simulink model "bicycle_model"  (R2018b)
settings: Solver=FixedStepAuto  StartTime=0.0  StopTime=10  FixedStep=0.001  RelTol=1e-3
values from neighbouring files (symbols this model uses):
  a = 1.8    [bicycle_coefficient_formula.m]    (also in bicycle_coefficient_roadcar.m = 1.1; formulacar_params.mat; roadcar_params.mat = 1.1)
  A = 1.25    [bicycle_coefficient_formula.m]    (also in bicycle_coefficient_roadcar.m = 1.8; formulacar_params.mat; roadcar_params.mat = 1.8)
  a1F = -1e-5    (= -1e-05)    [bicycle_coefficient_formula.m]    (also in bicycle_coefficient_roadcar.m; formulacar_params.mat; roadcar_params.mat)
  a1R = -1e-5    (= -1e-05)    [bicycle_coefficient_formula.m]    (also in bicycle_coefficient_roadcar.m; formulacar_params.mat; roadcar_params.mat)
  a2F = 1.25    [bicycle_coefficient_formula.m]    (also in bicycle_coefficient_roadcar.m = 0.95; formulacar_params.mat; roadcar_params.mat = 0.95)
  a2R = 1.25    [bicycle_coefficient_formula.m]    (also in bicycle_coefficient_roadcar.m = 0.95; formulacar_params.mat; roadcar_params.mat = 0.95)
  b = L-a    (= 1.7)    [bicycle_coefficient_formula.m]    (also in bicycle_coefficient_roadcar.m; formulacar_params.mat; roadcar_params.mat)
  BF = 0.2719    [bicycle_coefficient_formula.m]    (also in bicycle_coefficient_roadcar.m = 0.0813; formulacar_params.mat; roadcar_params.mat = 0.0813)
  BR = 0.3609    [bicycle_coefficient_formula.m]    (also in bicycle_coefficient_roadcar.m = 0.0925; formulacar_params.mat; roadcar_params.mat = 0.0925)
  CF = 1.8391    [bicycle_coefficient_formula.m]    (also in bicycle_coefficient_roadcar.m = 1.2947; formulacar_params.mat; roadcar_params.mat = 1.2947)
  CR = 1.7631    [bicycle_coefficient_formula.m]    (also in bicycle_coefficient_roadcar.m = 1.2617; formulacar_params.mat; roadcar_params.mat = 1.2617)
  cz = 1    [bicycle_coefficient_formula.m]    (also in bicycle_coefficient_roadcar.m = 0; formulacar_params.mat; roadcar_params.mat = 0)
  EF = -2.5276    [bicycle_coefficient_formula.m]    (also in bicycle_coefficient_roadcar.m = -8.3966; formulacar_params.mat; roadcar_params.mat = -8.3966)
  ER = -1.989    [bicycle_coefficient_formula.m]    (also in bicycle_coefficient_roadcar.m = -8.7012; formulacar_params.mat; roadcar_params.mat = -8.7012)
  g = 9.81    [bicycle_coefficient_formula.m]    (also in bicycle_coefficient_roadcar.m; formulacar_params.mat; roadcar_params.mat)
  I = 1500    [bicycle_coefficient_formula.m]    (also in bicycle_coefficient_roadcar.m = 3500; formulacar_params.mat; roadcar_params.mat = 3500)
  input = 1    [bicycle_script.m]    (also in formulacar_params.mat = 0; roadcar_params.mat = 0)
  L = 3.5    [bicycle_coefficient_formula.m]    (also in bicycle_coefficient_roadcar.m = 2.8; formulacar_params.mat; roadcar_params.mat = 2.8)
  m = 850    [bicycle_coefficient_formula.m]    (also in bicycle_coefficient_roadcar.m = 1650; formulacar_params.mat; roadcar_params.mat = 1650)
  rho = 1.225    [bicycle_coefficient_formula.m]    (also in bicycle_coefficient_roadcar.m; formulacar_params.mat; roadcar_params.mat)
  SA = 11    [bicycle_coefficient_formula.m]    (also in bicycle_coefficient_roadcar.m = 18; formulacar_params.mat; roadcar_params.mat = 18)
  slope = 2    [bicycle_coefficient_formula.m]    (also in bicycle_coefficient_roadcar.m; formulacar_params.mat; roadcar_params.mat)
  SR = 10    [bicycle_coefficient_formula.m]    (also in bicycle_coefficient_roadcar.m = 20; formulacar_params.mat; roadcar_params.mat = 20)
  V = 120    [bicycle_coefficient_formula.m]    (also in bicycle_coefficient_roadcar.m; formulacar_params.mat; roadcar_params.mat)
libraries: simulink_extras x5, simulink x1
settings Model: Creator=Cassio.Freitas  LastModifiedBy=Cassio.Freitas

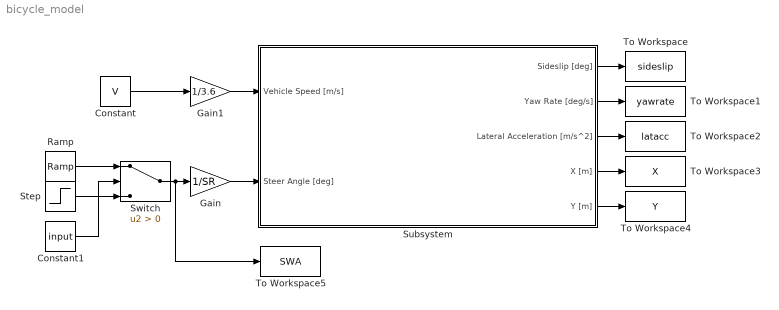
== system bicycle_model ==
  Constant : Constant  Value=V
  Constant1 : Constant  Value=input  SampleTime=0.01
  Gain : Gain  Gain=1/SR
  Gain1 : Gain  Gain=1/3.6
  Ramp : simulink/Sources/Ramp  slope=slope  start=0  InitialOutput=0
  Step : Step  Time=3  After=SA  SampleTime=0.001
  Subsystem : Subsystem
  Switch : Switch  Criteria=u2 > Threshold
  To Workspace : ToWorkspace  VariableName=sideslip  SaveFormat=Timeseries  SampleTime=-1
  To Workspace1 : ToWorkspace  VariableName=yawrate  SaveFormat=Timeseries  SampleTime=-1
  To Workspace2 : ToWorkspace  VariableName=latacc  SaveFormat=Timeseries  SampleTime=-1
  To Workspace3 : ToWorkspace  VariableName=X  SaveFormat=Timeseries  SampleTime=-1
  To Workspace4 : ToWorkspace  VariableName=Y  SaveFormat=Timeseries  SampleTime=-1
  To Workspace5 : ToWorkspace  VariableName=SWA  SaveFormat=Timeseries  SampleTime=-1
  wires:
  Subsystem/1(Sideslip [deg]) -> To Workspace/1
  Subsystem/2(Yaw Rate [deg/s]) -> To Workspace1/1
  Subsystem/3(Lateral Acceleration [m/s^2]) -> To Workspace2/1
  Subsystem/4(X [m]) -> To Workspace3/1
  Subsystem/5(Y [m]) -> To Workspace4/1
  Gain/1 -> Subsystem/2(Steer Angle [deg])
  Gain1/1 -> Subsystem/1(Vehicle Speed [m/s])
  Constant/1 -> Gain1/1
  Switch/1 -> To Workspace5/1, Gain/1
  Step/1 -> Switch/3
  Ramp/1 -> Switch/1
  Constant1/1 -> Switch/2

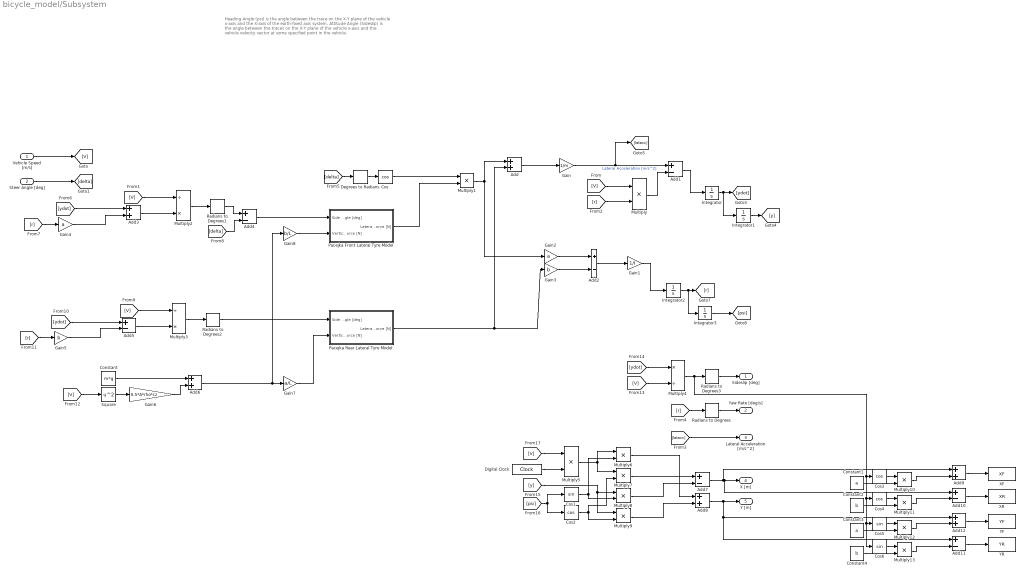
== system bicycle_model/Subsystem ==
  note: Heading Angle (psi) is the angle between the trace on the X-Y plane of the vehicle x-axis and the X-axis of the earth-fixed axis system.
      | Attitude Angle (Sideslip) is the angle between the traces on the X-Y plane of the vehicle x-axis and the vehicle velocity vector at some specified point in the vehicle.
  Vehicle Speed [m/s] : Inport
  Steer Angle [deg] : Inport  Port=2
  Add{,3,6,8..9,12} (6 alike) : Sum
  Add{1..2,4..5,7,10..11} (7 alike) : Sum  Inputs=+-
  Constant : Constant  Value=m*g
  Constant1 : Constant  Value=a
  Constant2 : Constant  Value=b
  Constant3 : Constant  Value=a
  Constant4 : Constant  Value=b
  Cos{,2..4} (4 alike) : Trigonometry  Operator=cos
  Cos1 : Trigonometry
  Cos5 : Trigonometry
  Cos6 : Trigonometry
  Degrees to Radians : simulink_extras/Transformations/Degrees to Radians
  Digital Clock : DigitalClock  SampleTime=0.001
  Gain : Gain  Gain=1/m
  Gain1 : Gain  Gain=1/I
  Gain2 : Gain  Gain=a
  Gain3 : Gain  Gain=b
  Gain4 : Gain  Gain=a
  Gain5 : Gain  Gain=b
  Gain6 : Gain  Gain=0.5*A*rho*cz
  Gain7 : Gain  Gain=a/L
  Gain8 : Gain  Gain=b/L
  Integrator{,1..3} (4 alike) : Integrator
  Multiply{,1,6..13} (10 alike) : Product
  Multiply2 : Product  Inputs=/*
  Multiply3 : Product  Inputs=/*
  Multiply4 : Product  Inputs=*/
  Multiply5 : Product  Inputs=**
  Pacejka Front Lateral Tyre Model : Subsystem
  Pacejka Rear Lateral Tyre Model : Subsystem
  Radians to Degrees{,1..3} (4 alike) : simulink_extras/Transformations/Radians to Degrees
  Square : Math  Operator=square  SaturateOnIntegerOverflow=on
  XF : ToWorkspace  VariableName=XF  SaveFormat=Timeseries  SampleTime=-1
  XR : ToWorkspace  VariableName=XR  SaveFormat=Timeseries  SampleTime=-1
  YF : ToWorkspace  VariableName=YF  SaveFormat=Timeseries  SampleTime=-1
  YR : ToWorkspace  VariableName=YR  SaveFormat=Timeseries  SampleTime=-1
  Sideslip [deg] : Outport
  Yaw Rate [deg/s] : Outport  Port=2
  Lateral Acceleration [m/s^2] : Outport  Port=3
  X [m] : Outport  Port=4
  Y [m] : Outport  Port=5
  wires:
  Vehicle Speed [m/s]/1 -> [V]
  Steer Angle [deg]/1 -> [delta]
  Add/1 -> Gain/1
  Gain/1 -> [latacc], Add1/1  "Lateral Acceleration [m/s^2]"
  Multiply/1 -> Add1/2
  [V] -> Multiply/1
  [r] -> Multiply/2
  Integrator/1 -> Integrator1/1, [ydot]
  Add1/1 -> Integrator/1
  Integrator1/1 -> [y]
  Gain1/1 -> Integrator2/1
  Add2/1 -> Gain1/1
  [latacc] -> Lateral Acceleration [m/s^2]/1
  Integrator2/1 -> Integrator3/1, [r]
  Integrator3/1 -> [psi]
  [r] -> Radians to Degrees/1
  Radians to Degrees/1 -> Yaw Rate [deg/s]/1
  Gain2/1 -> Add2/1
  Gain3/1 -> Add2/2
  Pacejka Front Lateral Tyre Model/1(Lateral Force [N]) -> Multiply1/2
  Multiply1/1 -> Gain2/1, Add/1
  Pacejka Rear Lateral Tyre Model/1(Lateral Force [N]) -> Add/2, Gain3/1
  [delta] -> Degrees to Radians/1
  Degrees to Radians/1 -> Cos/1
  Cos/1 -> Multiply1/1
  Add3/1 -> Multiply2/2
  [V] -> Multiply2/1
  [r] -> Gain4/1
  [ydot] -> Add3/1
  Gain4/1 -> Add3/2
  Multiply2/1 -> Radians to Degrees1/1
  [delta] -> Add4/2
  Radians to Degrees1/1 -> Add4/1
  Add4/1 -> Pacejka Front Lateral Tyre Model/1(Side Slip Angle [deg])
  [r] -> Gain5/1
  [V] -> Multiply3/1
  Radians to Degrees2/1 -> Pacejka Rear Lateral Tyre Model/1(Side Slip Angle [deg])
  Add5/1 -> Multiply3/2
  Multiply3/1 -> Radians to Degrees2/1
  Gain5/1 -> Add5/2
  [ydot] -> Add5/1
  [V] -> Square/1
  Square/1 -> Gain6/1
  Gain6/1 -> Add6/2
  Constant/1 -> Add6/1
  Add6/1 -> Gain8/1, Gain7/1
  Gain7/1 -> Pacejka Rear Lateral Tyre Model/2(Vertical Force [N])
  Gain8/1 -> Pacejka Front Lateral Tyre Model/2(Vertical Force [N])
  [V] -> Multiply4/2
  [ydot] -> Multiply4/1
  Radians to Degrees3/1 -> Sideslip [deg]/1
  Digital Clock/1 -> Multiply5/2
  [V] -> Multiply5/1
  [psi] -> Cos1/1, Cos2/1
  Multiply7/1 -> Add7/1
  Multiply8/1 -> Add7/2
  Multiply6/1 -> Add8/1
  Multiply9/1 -> Add8/2
  Multiply5/1 -> Multiply7/1, Multiply6/1
  [y] -> Multiply9/1, Multiply8/1
  Cos1/1 -> Multiply8/2, Multiply6/2
  Cos2/1 -> Multiply7/2, Multiply9/2
  Add7/1 -> Add10/1, X [m]/1, Add9/1
  Multiply10/1 -> Add9/2
  Constant1/1 -> Multiply10/2
  Cos3/1 -> Multiply10/1
  Cos4/1 -> Multiply11/1
  Multiply11/1 -> Add10/2
  Multiply4/1 -> Cos6/1, Cos5/1, Cos4/1, Cos3/1, Radians to Degrees3/1
  Constant2/1 -> Multiply11/2
  Constant4/1 -> Multiply13/2
  Multiply13/1 -> Add11/2
  Add8/1 -> Add11/1, Add12/1, Y [m]/1
  Cos6/1 -> Multiply13/1
  Cos5/1 -> Multiply12/1
  Multiply12/1 -> Add12/2
  Constant3/1 -> Multiply12/2
  Add9/1 -> XF/1
  Add10/1 -> XR/1
  Add12/1 -> YF/1
  Add11/1 -> YR/1

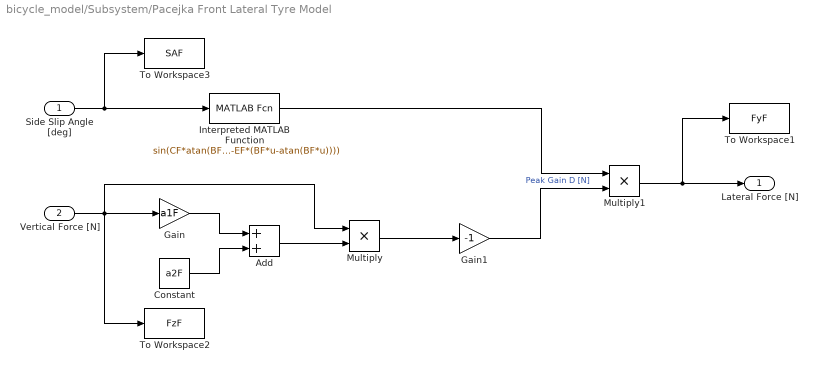
== system bicycle_model/Subsystem/Pacejka Front Lateral Tyre Model ==
  Side Slip Angle [deg] : Inport
  Vertical Force [N] : Inport  Port=2
  Add : Sum
  Constant : Constant  Value=a2F
  Gain : Gain  Gain=a1F
  Gain1 : Gain  Gain=-1
  Interpreted MATLAB Function : MATLABFcn  MATLABFcn=sin(CF*atan(BF*u-EF*(BF*u-atan(BF*u))))
  Multiply : Product
  Multiply1 : Product
  To Workspace1 : ToWorkspace  VariableName=FyF  SaveFormat=Timeseries  SampleTime=-1
  To Workspace2 : ToWorkspace  VariableName=FzF  SaveFormat=Timeseries  SampleTime=-1
  To Workspace3 : ToWorkspace  VariableName=SAF  SaveFormat=Timeseries  SampleTime=-1
  Lateral Force [N] : Outport
  wires:
  Vertical Force [N]/1 -> To Workspace2/1, Gain/1, Multiply/1
  Constant/1 -> Add/2
  Gain/1 -> Add/1
  Add/1 -> Multiply/2
  Multiply/1 -> Gain1/1
  Gain1/1 -> Multiply1/2  "Peak Gain D [N]"
  Side Slip Angle [deg]/1 -> To Workspace3/1, Interpreted MATLAB Function/1
  Interpreted MATLAB Function/1 -> Multiply1/1
  Multiply1/1 -> To Workspace1/1, Lateral Force [N]/1

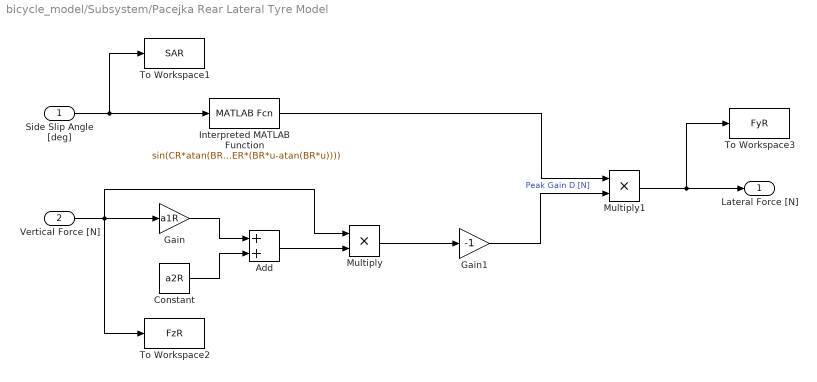
== system bicycle_model/Subsystem/Pacejka Rear Lateral Tyre Model ==
  Side Slip Angle [deg] : Inport
  Vertical Force [N] : Inport  Port=2
  Add : Sum
  Constant : Constant  Value=a2R
  Gain : Gain  Gain=a1R
  Gain1 : Gain  Gain=-1
  Interpreted MATLAB Function : MATLABFcn  MATLABFcn=sin(CR*atan(BR*u-ER*(BR*u-atan(BR*u))))
  Multiply : Product
  Multiply1 : Product
  To Workspace1 : ToWorkspace  VariableName=SAR  SaveFormat=Timeseries  SampleTime=-1
  To Workspace2 : ToWorkspace  VariableName=FzR  SaveFormat=Timeseries  SampleTime=-1
  To Workspace3 : ToWorkspace  VariableName=FyR  SaveFormat=Timeseries  SampleTime=-1
  Lateral Force [N] : Outport
  wires:
  Interpreted MATLAB Function/1 -> Multiply1/1
  Side Slip Angle [deg]/1 -> To Workspace1/1, Interpreted MATLAB Function/1
  Gain1/1 -> Multiply1/2  "Peak Gain D [N]"
  Multiply/1 -> Gain1/1
  Add/1 -> Multiply/2
  Gain/1 -> Add/1
  Constant/1 -> Add/2
  Vertical Force [N]/1 -> Multiply/1, To Workspace2/1, Gain/1
  Multiply1/1 -> To Workspace3/1, Lateral Force [N]/1
